simulink model "first_order_open_and_closed_loop"  (R2015a)
settings: Solver=ode45  StartTime=0.0  StopTime=10.0  RelTol=1e-3
libraries: simulink_extras x4, powerlib x1
settings Model: Creator=chand  LastModifiedBy=chand

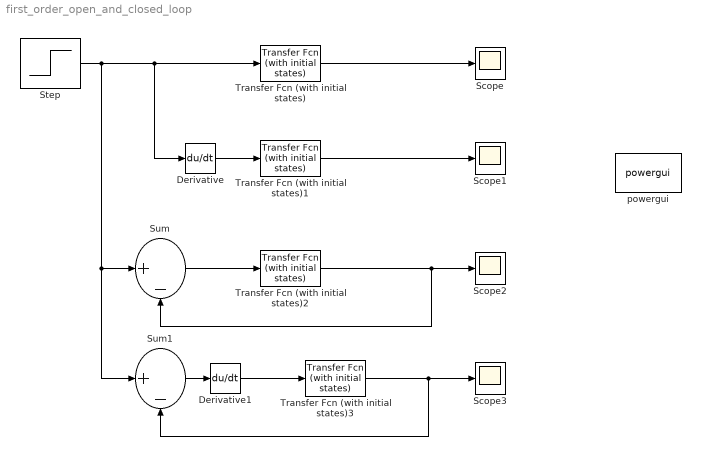
== system first_order_open_and_closed_loop ==
  Derivative : Derivative
  Derivative1 : Derivative
  Scope{,1..3} (4 alike) : Scope
      Scope2 settings: SaveName=ScopeData2
      Scope3 settings: SaveName=ScopeData3
  Step : Step  Time=0  After=10  SampleTime=0
  Sum : Sum  Inputs=|+-
  Sum1 : Sum  Inputs=|+-
  Transfer Fcn (with initial states){,1..3} (4 alike) : simulink_extras/Additional Linear/Transfer Fcn (with initial states)  N=[4]  D="[1  2]"  X0=0
  powergui : powerlib/powergui  Priority=1  SimulationMode=Continuous  SolverType=Tustin/Backward Euler (TBE)  SampleTime=50e-6  frequency=60  SPID=off  DisableSnubberDevices=off  DisableRonSwitches=off  DisableVfSwitches=off  SwTol=0  DisplayEquations=off  Interpol=off  methode=off  Ts=100  FunctionMessages=off  echomessages=off  HookPort=off  EnableUseOfTLC=off  x0status=blocks  frequencyindice=60  Pbase=100e6  ErrMax=1e-4  Iterations=50  UnitsV=kV  UnitsW=MW  buscounter=0  RestoreLinks=warning  ResistiveCurrentMeasurement=off  Frange=[0:2:500]  Ylog=off  Xlog=on  ShowGrid=off  save=off  variable=ZData  structure=0  ZoomFFT=off  StartTime=0.0  cycles=1  DisplayStyle=1  fundamental=60  FreqAxis=off  MaxFrequency=1000  frequencyindicesteady=1  RmsSteady=1  display=off
  wires:
  Step/1 -> Sum1/1, Sum/1, Derivative/1, Transfer Fcn (with initial states)/1
  Transfer Fcn (with initial states)/1 -> Scope/1
  Derivative/1 -> Transfer Fcn (with initial states)1/1
  Transfer Fcn (with initial states)1/1 -> Scope1/1
  Sum/1 -> Transfer Fcn (with initial states)2/1
  Transfer Fcn (with initial states)2/1 -> Sum/2, Scope2/1
  Derivative1/1 -> Transfer Fcn (with initial states)3/1
  Transfer Fcn (with initial states)3/1 -> Scope3/1, Sum1/2
  Sum1/1 -> Derivative1/1
